simulink model "test_full_set"  (Simulink 8.8)
settings: Solver=FixedStepDiscrete  StartTime=0.0  StopTime=10  FixedStep=0.01  RelTol=1e-3  EnableMultiTasking=on
InitFcn:
  | px4_ap1_mdl_callback('check_model');
undefined symbols (not defined in the file or in its folder): s
libraries: px4_ap1_color_power_led_lib x1, px4_ap1_mpu_6000_lib x1, px4_ap1_pwm_aux_out_lib x1, px4_ap1_pwm_main_out_lib x1, px4_ap1_px4setup_lib x1, px4_ap1_fmu_amber_led_lib x1, px4_ap1_gps_lib x1, px4_ap1_hmc5883_lib x1, px4_ap1_ms5611_lib x1, px4_ap1_sdcard_logger_lib x1, px4_ap1_signal_output_lib x1, px4_ap1_rc_ppm_input_lib x1
settings Model: Creator=Privat  LastModifiedBy=Privat
settings OptimizationCC: ExpressionDepthLimit=2147483647  InitFltsAndDblsToZero=on  LifeSpan=1
settings DebuggingCC: SolverPrmCheckMsg=warning  InheritedTsInSrcMsg=none
settings HardwareCC: ProdLargestAtomicInteger=Long  ProdLargestAtomicFloat=Float  ProdEndianess=LittleEndian  ProdHWDeviceType=ARM Compatible->ARM 7
settings SFSimCC: SimParseCustomCode=off
settings RTWCC: SystemTargetFile=px4_ap1.tlc  GenCodeOnly=on  GenerateMakefile=off
settings CodeAppCC: IgnoreCustomStorageClasses=off  CustomSymbolStrType=$N$R$M  InternalIdentifier=Classic
settings STFCustomTargetCC: TargetLangStandard=C99 (ISO)  ModelReferenceCompliant=off  IncludeMdlTerminateFcn=off  CombineOutputUpdateFcns=on  ERTCustomFileBanners=on  SupportContinuousTime=off  SupportNonInlinedSFcns=off  RemoveResetFunc=on  MATLABClassNameForMDSCustomization=Simulink.SoftwareTarget.ERTCustomization  CPPClassGenCompliant=on  GRTInterface=off  SystemTargetFile=px4_ap1.tlc
settings ERTTargetCC: TargetLangStandard=C99 (ISO)  MultiwordLength=2048  ModelReferenceCompliant=off  ParMdlRefBuildCompliant=off  CompOptLevelCompliant=off  ConcurrentExecutionCompliant=off  IncludeMdlTerminateFcn=off  ERTFirstTimeCompliant=off  ModelStepFunctionPrototypeControlCompliant=off  UseToolchainInfoCompliant=off  ERTSrcFileBannerTemplate=px4_ap1_code_template.cgt  ERTHdrFileBannerTemplate=px4_ap1_code_template.cgt  ERTDataSrcFileTemplate=px4_ap1_code_template.cgt  ERTDataHdrFileTemplate=px4_ap1_code_template.cgt  ERTCustomFileTemplate=px4_ap1_main.tlc  ConvertIfToSwitch=off  SuppressUnreachableDefaultCases=off

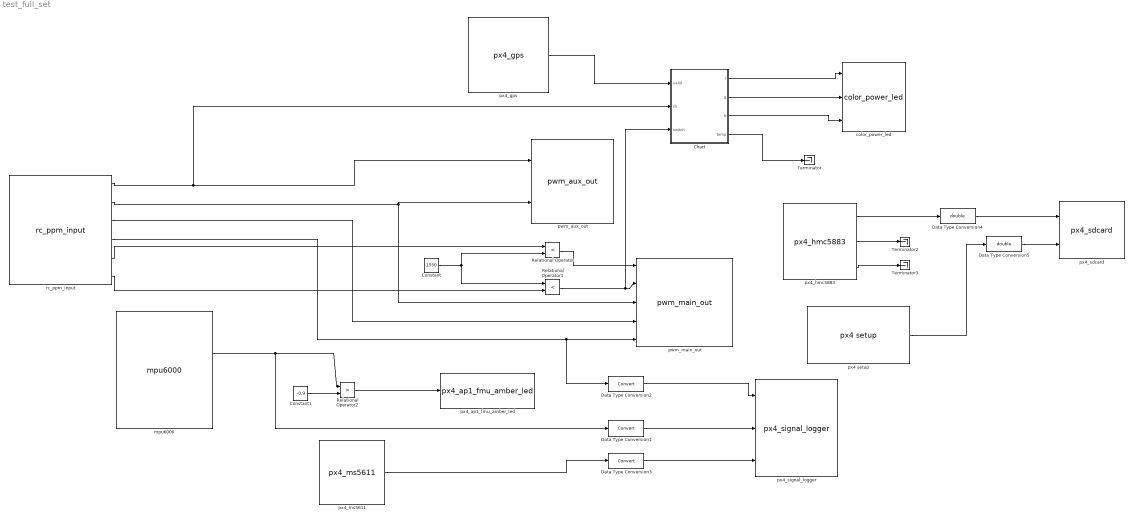
== system test_full_set ==
  Chart : Stateflow chart  TreatAsAtomicUnit=on
  Constant : Constant  Value=1550
  Constant1 : Constant  Value=-0.9
  Data Type Conversion1 : DataTypeConversion
  Data Type Conversion2 : DataTypeConversion
  Data Type Conversion3 : DataTypeConversion
  Data Type Conversion4 : DataTypeConversion  OutDataTypeStr=double
  Data Type Conversion5 : DataTypeConversion  OutDataTypeStr=double
  Relational Operator : RelationalOperator  Operator=<  OutDataTypeStr=boolean  RndMeth=Nearest
  Relational Operator1 : RelationalOperator  Operator=<  OutDataTypeStr=boolean  RndMeth=Nearest
  Relational Operator2 : RelationalOperator  Operator=>  RndMeth=Nearest
  Terminator : Terminator
  Terminator2 : Terminator
  Terminator3 : Terminator
  color_power_led : px4_ap1_color_power_led_lib/color_power_led
  mpu6000 : px4_ap1_mpu_6000_lib/mpu6000  Description=Setup for PX4 native software  accelRange=+/- 2g  gyroRange=250°/s  filter=5Hz  accXcorr=1  accYcorr=1  accZcorr=1  accXoff=0  accYoff=0  accZoff=0
  pwm_aux_out : px4_ap1_pwm_aux_out_lib/pwm_aux_out  Description=Setup for PX4 native software  aux1=on  aux2=off  aux3=off  aux4=off  aux5=on  aux6=off  pwm_1_4=115  pwm_5_6=311
  pwm_main_out : px4_ap1_pwm_main_out_lib/pwm_main_out  Description=Setup for PX4 native software  main1=on  main2=off  main3=on  main4=off  main5=on  main6=off  main7=off  main8=off  def_pwm=222  alt_pwm=111  pwm_1_2=Default  pwm_3_4=Alternate  pwm_5_8=Default
  px4 setup : px4_ap1_px4setup_lib/px4 setup  SampleTimeValue=0.01  cbBuild=on  cbUpload=on  cbPort=COM3  cpuLoad=on  debugmode=on
  px4_ap1_fmu_amber_led : px4_ap1_fmu_amber_led_lib/px4_ap1_fmu_amber_led  Description=TODO
  px4_gps : px4_ap1_gps_lib/px4_gps  Description=Setup for PX4 native software  baud=9600  latlon=off  speed=off  course=off  time=off  date=off
  px4_hmc5883 : px4_ap1_hmc5883_lib/px4_hmc5883  Description=Setup for PX4 native software  magRange=+/- 1.3Ga
  px4_ms5611 : px4_ap1_ms5611_lib/px4_ms5611  Description=Setup for PX4 native software
  px4_sdcard : px4_ap1_sdcard_logger_lib/px4_sdcard  Description=Setup for PX4 native software  sampleTime=0.5  sigCnt=2
  px4_signal_logger : px4_ap1_signal_output_lib/px4_signal_logger  Description=Setup for PX4 native software  sampleTime=500  sigCnt=3
  rc_ppm_input : px4_ap1_rc_ppm_input_lib/rc_ppm_input  Description=Setup for PX4 native software  ch1=on  ch2=on  ch3=on  ch4=on  ch5=on  ch6=on  ch7=off  ch8=off  ch9=off  ch10=off  ch11=off  ch12=off  ch13=off  ch14=off  ch15=off  ch16=off  ch17=off  ch18=off
  wires:
  rc_ppm_input/1 -> pwm_aux_out/1, Chart/2(ch)
  rc_ppm_input/2 -> pwm_aux_out/2, pwm_main_out/3
  rc_ppm_input/3 -> pwm_main_out/4
  rc_ppm_input/4 -> pwm_main_out/5, Data Type Conversion2/1
  Constant/1 -> Relational Operator1/1, Relational Operator/2
  Relational Operator1/1 -> pwm_main_out/2, Chart/3(switch)
  rc_ppm_input/6 -> Relational Operator1/2
  rc_ppm_input/5 -> Relational Operator/1
  Relational Operator/1 -> pwm_main_out/1
  Constant1/1 -> Relational Operator2/2
  Relational Operator2/1 -> px4_ap1_fmu_amber_led/1
  mpu6000/3 -> Relational Operator2/1, Data Type Conversion1/1
  px4_gps/1 -> Chart/1(valid)
  Data Type Conversion1/1 -> px4_signal_logger/2
  Data Type Conversion2/1 -> px4_signal_logger/1
  Chart/1(r) -> color_power_led/1
  Chart/2(g) -> color_power_led/2
  Chart/3(b) -> color_power_led/3
  Chart/4(temp) -> Terminator/1
  px4_ms5611/1 -> Data Type Conversion3/1
  Data Type Conversion3/1 -> px4_signal_logger/3
  px4_hmc5883/1 -> Data Type Conversion4/1
  px4_hmc5883/2 -> Terminator2/1
  px4_hmc5883/3 -> Terminator3/1
  Data Type Conversion4/1 -> px4_sdcard/1
  px4 setup/1 -> Data Type Conversion5/1
  Data Type Conversion5/1 -> px4_sdcard/2

== stateflow chart Chart ==
  (default) -> (junction 10)
  (junction 10) -> (junction 11) [order 1] : [switch == 0]
  (junction 11) -> (junction 12) [order 1] : [valid == 1]
      | {r = 0; g = 255; b = 0;}
  (junction 12) -> (junction 14)
  (junction 10) -> (junction 15) [order 2]
  (junction 11) -> (junction 13) [order 2]
  (junction 13) -> (junction 14) : {r = 255; g = 255; b = 255;}
  (junction 14) -> (junction 16)
  (junction 15) -> (junction 16) : {r = 0;
      | g = 0;
      | temp = (ch - 1000) * 255 / 1000;
      | b = temp;}
  data: r output uint8; g output uint8; b output uint8; valid input double; ch input double; switch input double; temp output single
